simulink model "CTRL_TRGT_UG_test"  (R2023b)
settings: Solver=VariableStepAuto  StartTime=0.0  StopTime=10.0  RelTol=1e-3
libraries: CTRL_TRGT_UG x1
settings Model: Creator=blatak  LastModifiedBy=blatak

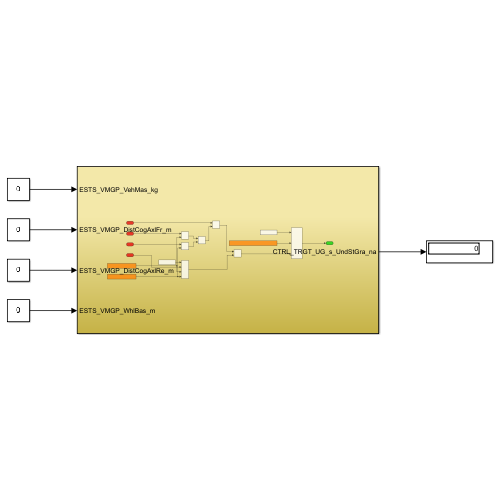
[thumbnail: Simulink's stored preview of the top-level diagram]
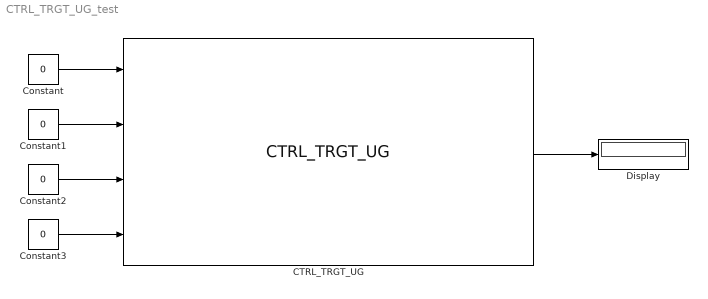
== system CTRL_TRGT_UG_test ==
  CTRL_TRGT_UG : CTRL_TRGT_UG/CTRL_TRGT_UG  SystemSampleTime=-1  VariantActivationTime=update diagram  AllowFlexibleInterface=on  Latency=0  AutoFrameSizeCalculation=off
  Constant{,1..3} (4 alike) : Constant  Value=0  OutDataTypeStr=single
  Display : Display
  wires:
  Constant/1 -> CTRL_TRGT_UG/1
  Constant1/1 -> CTRL_TRGT_UG/2
  Constant2/1 -> CTRL_TRGT_UG/3
  Constant3/1 -> CTRL_TRGT_UG/4
  CTRL_TRGT_UG/1 -> Display/1
